simulink model "adrcControllerModel"  (R2021a)
settings: Solver=VariableStepAuto  StartTime=0.0  StopTime=10.0  RelTol=1e-3
settings Model: Creator=krzys  LastModifiedBy=krzys

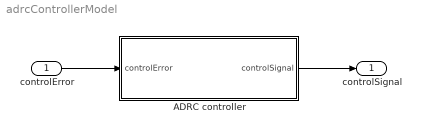
== system adrcControllerModel ==
  controlError : Inport
  ADRC controller : Subsystem  mask{dynamicsOrder=2, inputGainParameter=3, controllerBandwidth=4, observerBandwidth=5}
      mask prompts: dynamicsOrder "Dynamics order:"; inputGainParameter "Input gain parameter:"; controllerBandwidth "Controller bandwidth:"; observerBandwidth "Observer bandwidth:"
      mask TypeOptions dynamicsOrder: Dynamics order/Value
      mask TypeOptions inputGainParameter: Input gain parameter/Value
      mask TypeOptions controllerBandwidth: Controller bandwidth/Value
      mask TypeOptions observerBandwidth: Observer bandwidth/Value
  controlSignal : Outport
  wires:
  controlError/1 -> ADRC controller/1(controlError)
  ADRC controller/1(controlSignal) -> controlSignal/1

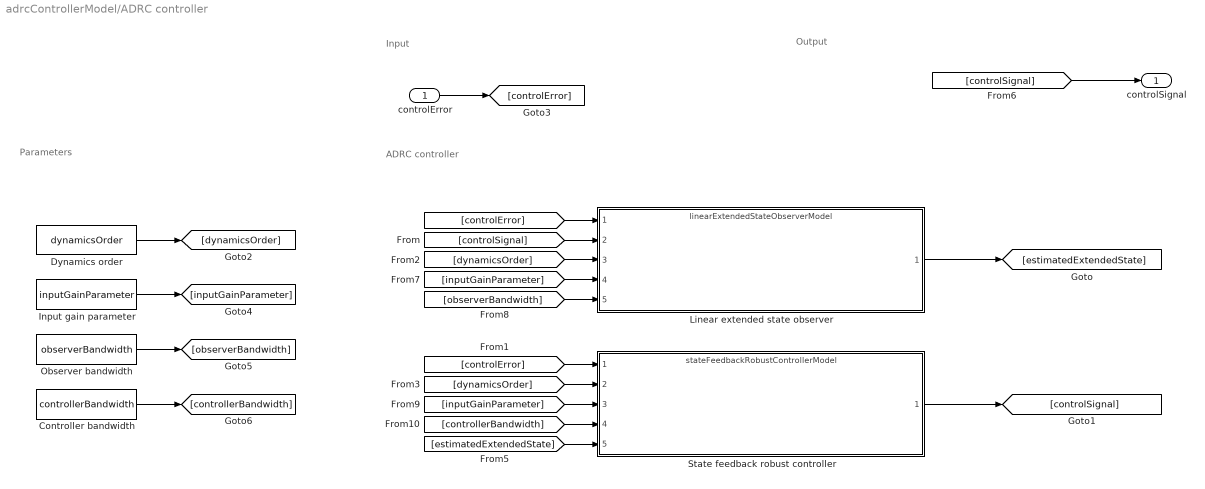
== system adrcControllerModel/ADRC controller ==
  note: ADRC controller
  note: Output
  note: Input
  note: Parameters
  controlError : Inport
  Controller bandwidth : Constant  Value=controllerBandwidth
  Dynamics order : Constant  Value=dynamicsOrder
  Input gain parameter : Constant  Value=inputGainParameter
  Linear extended state observer : ModelReference  ModelNameDialog=linearExtendedStateObserverModel.slx  SimulationMode=Normal  ModelReferenceVersion=1.23
  Observer bandwidth : Constant  Value=observerBandwidth
  State feedback robust controller : ModelReference  ModelNameDialog=stateFeedbackRobustControllerModel.slx  SimulationMode=Normal  ModelReferenceVersion=1.13
  controlSignal : Outport
  wires:
  [dynamicsOrder] -> Linear extended state observer/3
  Linear extended state observer/1 -> [estimatedExtendedState]
  Input gain parameter/1 -> [inputGainParameter]
  [controllerBandwidth] -> State feedback robust controller/4
  [dynamicsOrder] -> State feedback robust controller/2
  [controlSignal] -> controlSignal/1
  [controlError] -> Linear extended state observer/1
  [controlSignal] -> Linear extended state observer/2
  State feedback robust controller/1 -> [controlSignal]
  [inputGainParameter] -> State feedback robust controller/3
  Observer bandwidth/1 -> [observerBandwidth]
  [estimatedExtendedState] -> State feedback robust controller/5
  [inputGainParameter] -> Linear extended state observer/4
  [controlError] -> State feedback robust controller/1
  [observerBandwidth] -> Linear extended state observer/5
  controlError/1 -> [controlError]
  Dynamics order/1 -> [dynamicsOrder]
  Controller bandwidth/1 -> [controllerBandwidth]
